simulink library "lib_controller"  (R2015a)
settings: Solver=ode45  StartTime=0.0  StopTime=10.0  RelTol=1e-3
values from neighbouring files (symbols this model uses):
  CG_0 = [0,0,0.02]'    [SetupComplete.m]
  g = 9.81    [SetupComplete.m]
  h_M = 0.064    [SetupComplete.m]
  I_BAC_0 = [ Ix,0,Ixz;0,Iy,0;Ixz,0,Iz]    [SetupComplete.m]
  l = 0.3450    (= 0.345)    [NDI_components.m]    (also in SetupComplete.m; robust_controller.m)
  m = 3.51    [SetupComplete.m]
  m_0 = 2.61    [SetupComplete.m]
  m_M = 0.300    (= 0.3)    [SetupComplete.m]
  T_sim = 0.01    [Run3Copter.m]
undefined symbols (not defined in the file or in its folder): Theta_1_roll_last, Theta_2_roll_last, Theta_3_roll_last, V_long_lastA_w_z, V_long_lastAoA, V_roll_last, V_yaw_last, W_long_lastA_w_z, W_long_lastAoA, W_roll_last, W_yaw_last
libraries: simulink x65, Adaptive_FaultTolerantControl x8, lib_controller x5, qcatlib x4, dspinverses x4, aerolibtransform2 x3, aerolib6dofsys x1
(part 5 of 10)

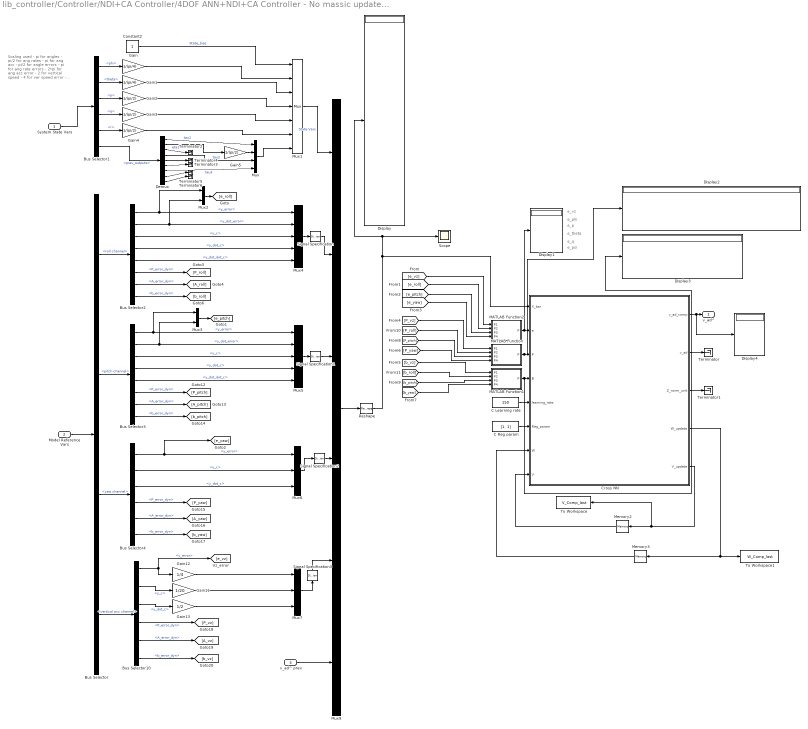
== system lib_controller/Controller/NDI+CA Controller/4DOF ANN+NDI+CA Controller - No massic update/Adaptive NN/Crossed NN ==
  note: e_vz
  note: Scaling used
      | - pi for angles
      | - pi/2 for ang rates
      | - pi for ang acc
      | - pi/2 for angle errors
      | - pi for ang rate errors
      | - 2*pi for ang acc error
      |
      | - 2 for vertical speed
      | - 4 for ver speed error
      | - 12 for vertical acc
      | - 18 for vertical acc error
  note: e_phi
  note: e_p
  note: e_theta
  note: e_q
  note: e_psi
  System State Vars : Inport
  Model Reference Vars : Inport  Port=2
  v_ad^ prev : Inport  Port=3
  Bus Selector : BusSelector  OutputSignals=roll channel,pitch channel,yaw channel,vertical acc channel
  Bus Selector1 : BusSelector  OutputSignals=phi,theta,p,q,r,prev_outputs
  Bus Selector10 : BusSelector  OutputSignals=y_error,y_c,y_dot_c,P_error_dyn,A_error_dyn,b_error_dyn
  Bus Selector2 : BusSelector  OutputSignals=y_error,y_dot_error,y_c,y_dot_c,y_dot_dot_c,P_error_dyn,A_error_dyn,b_error_dyn
  Bus Selector3 : BusSelector  OutputSignals=y_error,y_dot_error,y_c,y_dot_c,y_dot_dot_c,P_error_dyn,A_error_dyn,b_error_dyn
  Bus Selector4 : BusSelector  OutputSignals=y_error,y_c,y_dot_c,P_error_dyn,A_error_dyn,b_error_dyn
  C Learning rate : Constant  Value=150  SampleTime=T_sim
  C Reg param : Constant  Value=[1, 1]  SampleTime=T_sim
  Constant2 : Constant
  Cross NN : MATLAB Function  TreatAsAtomicUnit=on
  Demux : Demux  Outputs=9
  Display{,1..4} (5 alike) : Display
  Gain : Gain  Gain=1/(pi/4)
  Gain1 : Gain  Gain=1/(pi/4)
  Gain11 : Gain  Gain=1/20
  Gain12 : Gain  Gain=1/4
  Gain13 : Gain  Gain=1/2
  Gain{2..5} (4 alike) : Gain  Gain=1/(pi/2)
  MATLAB Function : MATLAB Function  TreatAsAtomicUnit=on
  MATLAB Function1 : MATLAB Function  TreatAsAtomicUnit=on
  MATLAB Function2 : MATLAB Function  TreatAsAtomicUnit=on
  Memory2 : Memory
  Memory3 : Memory
  Mux : Mux
  Mux1 : Mux  Inputs=7
  Mux2 : Mux  Inputs=2
  Mux3 : Mux  Inputs=2
  Mux4 : Mux  Inputs=5
  Mux5 : Mux  Inputs=5
  Mux6 : Mux  Inputs=3
  Mux7 : Mux  Inputs=3
  Mux9 : Mux  Inputs=6
  Reshape : Reshape
  Scope : Scope
      settings: SaveName=ScopeData8
  Signal Specification : SignalSpecification  Dimensions=5
  Signal Specification1 : SignalSpecification  Dimensions=5
  Signal Specification2 : SignalSpecification  Dimensions=3
  Signal Specification3 : SignalSpecification  Dimensions=3
  Terminator{,1..6} (7 alike) : Terminator
  To Workspace : ToWorkspace  VariableName=V_Comp_last  SampleTime=-1
      settings: MaxDataPoints=1
  To Workspace1 : ToWorkspace  VariableName=W_Comp_last  SampleTime=-1
      settings: MaxDataPoints=1
  v_ad^ : Outport
  wires:
  Cross NN/4(W_update) -> To Workspace1/1, Memory3/1
  Cross NN/5(V_update) -> Memory2/1, To Workspace/1
  Cross NN/2(v_ad) -> Terminator/1
  Memory3/1 -> Cross NN/7(W)
  Memory2/1 -> Cross NN/8(V)
  Cross NN/1(v_ad_comp) -> Display4/1, v_ad^/1
  C Learning rate/1 -> Cross NN/5(learning_rate)
  C Reg param/1 -> Cross NN/6(Reg_param)
  Cross NN/3(Z_norm_unit) -> Terminator1/1
  Mux9/1 -> Reshape/1
  Model Reference Vars/1 -> Bus Selector/1
  System State Vars/1 -> Bus Selector1/1
  Bus Selector1/1 -> Gain/1  "<phi>"
  Bus Selector1/2 -> Gain1/1  "<theta>"
  Bus Selector1/3 -> Gain2/1  "<p>"
  Bus Selector1/4 -> Gain3/1  "<q>"
  Bus Selector1/5 -> Gain4/1  "<r>"
  Bus Selector1/6 -> Demux/1  "<prev_outputs>"
  Gain5/1 -> Mux/2
  Mux1/1 -> Mux9/1  "State Vars"
  Mux/1 -> Mux1/7
  Gain2/1 -> Mux1/4
  Gain1/1 -> Mux1/3
  Gain3/1 -> Mux1/5
  Gain/1 -> Mux1/2
  Gain4/1 -> Mux1/6
  Constant2/1 -> Mux1/1  "State_bias"
  Bus Selector/1 -> Bus Selector2/1  "<roll channel>"
  Bus Selector2/1 -> Mux4/1, Mux2/1  "<y_error>"
  Bus Selector2/2 -> Mux4/2, Mux2/2  "<y_dot_error>"
  Bus Selector2/3 -> Mux4/3  "<y_c>"
  Bus Selector2/4 -> Mux4/4  "<y_dot_c>"
  Bus Selector2/5 -> Mux4/5  "<y_dot_dot_c>"
  Bus Selector/2 -> Bus Selector3/1  "<pitch channel>"
  Bus Selector3/1 -> Mux5/1, Mux3/1  "<y_error>"
  Bus Selector3/2 -> Mux5/2, Mux3/2  "<y_dot_error>"
  Bus Selector/3 -> Bus Selector4/1  "<yaw channel>"
  Bus Selector/4 -> Bus Selector10/1  "<vertical acc channel>"
  Bus Selector4/1 -> Mux6/1, [e_yaw]  "<y_error>"
  Mux2/1 -> [e_roll]
  Mux3/1 -> [e_pitch]
  Bus Selector2/6 -> [P_roll]  "<P_error_dyn>"
  Bus Selector2/7 -> [A_roll]  "<A_error_dyn>"
  Bus Selector2/8 -> [b_roll]  "<b_error_dyn>"
  Bus Selector10/1 -> Gain12/1, [e_vz]  "<y_error>"
  Bus Selector3/6 -> [P_pitch]  "<P_error_dyn>"
  Bus Selector3/7 -> [A_pitch]  "<A_error_dyn>"
  Bus Selector3/8 -> [b_pitch]  "<b_error_dyn>"
  Bus Selector4/4 -> [P_yaw]  "<P_error_dyn>"
  Bus Selector4/5 -> [A_yaw]  "<A_error_dyn>"
  Bus Selector4/6 -> [b_yaw]  "<b_error_dyn>"
  Bus Selector10/4 -> [P_vz]  "<P_error_dyn>"
  Bus Selector10/5 -> [A_vz]  "<A_error_dyn>"
  Bus Selector10/6 -> [b_vz]  "<b_error_dyn>"
  Bus Selector3/3 -> Mux5/3  "<y_c>"
  Bus Selector3/4 -> Mux5/4  "<y_dot_c>"
  Bus Selector3/5 -> Mux5/5  "<y_dot_dot_c>"
  Bus Selector4/2 -> Mux6/2  "<y_c>"
  Bus Selector4/3 -> Mux6/3  "<y_dot_c>"
  Bus Selector10/2 -> Gain11/1  "<y_c>"
  Bus Selector10/3 -> Gain13/1  "<y_dot_c>"
  v_ad^ prev/1 -> Mux9/6
  Reshape/1 -> Cross NN/1(X_bar), Display/1, Scope/1
  Mux5/1 -> Signal Specification1/1
  Gain12/1 -> Mux7/1
  Gain13/1 -> Mux7/3
  Gain11/1 -> Mux7/2
  Mux7/1 -> Signal Specification3/1
  MATLAB Function/1(P) -> Display2/1, Cross NN/3(P)
  [P_yaw] -> MATLAB Function/4(P4)
  [P_pitch] -> MATLAB Function/3(P3)
  [P_roll] -> MATLAB Function/2(P2)
  [P_vz] -> MATLAB Function/1(P1)
  MATLAB Function1/1(P) -> Display3/1, Cross NN/4(B)
  [b_vz] -> MATLAB Function1/1(P1)
  [b_roll] -> MATLAB Function1/2(P2)
  [b_pitch] -> MATLAB Function1/3(P3)
  [b_yaw] -> MATLAB Function1/4(P4)
  Demux/1 -> Mux/1  "tau1"
  Demux/2 -> Gain5/1  "eta1"
  Demux/4 -> Mux/3  "tau2"
  Demux/7 -> Mux/4  "tau3"
  Demux/3 -> Terminator2/1
  Demux/5 -> Terminator4/1
  Demux/6 -> Terminator3/1
  Demux/8 -> Terminator5/1
  Demux/9 -> Terminator6/1
  [e_yaw] -> MATLAB Function2/4(P4)
  [e_pitch] -> MATLAB Function2/3(P3)
  [e_roll] -> MATLAB Function2/2(P2)
  [e_vz] -> MATLAB Function2/1(P1)
  MATLAB Function2/1(P) -> Display1/1, Cross NN/2(e)
  Mux4/1 -> Signal Specification/1
  Signal Specification/1 -> Mux9/2
  Signal Specification1/1 -> Mux9/3
  Signal Specification2/1 -> Mux9/4
  Mux6/1 -> Signal Specification2/1
  Signal Specification3/1 -> Mux9/5

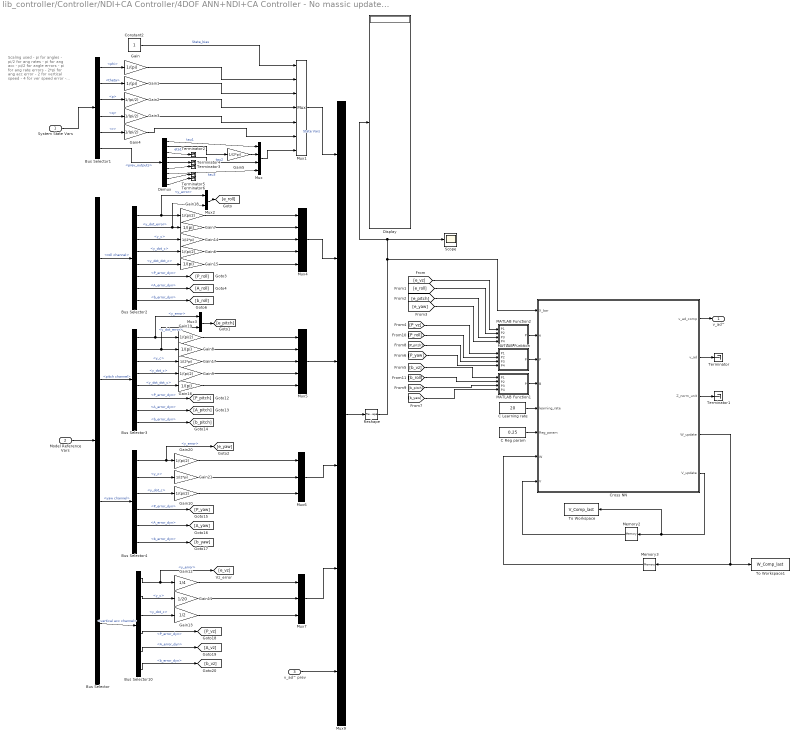
== system lib_controller/Controller/NDI+CA Controller/4DOF ANN+NDI+CA Controller - No massic update/Adaptive NN1/Complete crossed On-line (adaptive) multi-layer NN: AoA ==
  note: Scaling used
      | - pi for angles
      | - pi/2 for ang rates
      | - pi for ang acc
      | - pi/2 for angle errors
      | - pi for ang rate errors
      | - 2*pi for ang acc error
      |
      | - 2 for vertical speed
      | - 4 for ver speed error
      | - 12 for vertical acc
      | - 18 for vertical acc error
  System State Vars : Inport
  Model Reference Vars : Inport  Port=2
  v_ad^ prev : Inport  Port=3
  Bus Selector : BusSelector  OutputSignals=roll channel,pitch channel,yaw channel,vertical acc channel
  Bus Selector1 : BusSelector  OutputSignals=phi,theta,p,q,r,prev_outputs
  Bus Selector10 : BusSelector  OutputSignals=y_error,y_c,y_dot_c,P_error_dyn,A_error_dyn,b_error_dyn
  Bus Selector2 : BusSelector  OutputSignals=y_error,y_dot_error,y_c,y_dot_c,y_dot_dot_c,P_error_dyn,A_error_dyn,b_error_dyn
  Bus Selector3 : BusSelector  OutputSignals=y_error,y_dot_error,y_c,y_dot_c,y_dot_dot_c,P_error_dyn,A_error_dyn,b_error_dyn
  Bus Selector4 : BusSelector  OutputSignals=y_error,y_c,y_dot_c,P_error_dyn,A_error_dyn,b_error_dyn
  C Learning rate : Constant  Value=20  SampleTime=T_sim
  C Reg param : Constant  Value=0.25  SampleTime=T_sim
  Constant2 : Constant
  Cross NN : MATLAB Function  TreatAsAtomicUnit=on
  Demux : Demux  Outputs=9
  Display : Display
  Gain{,1,7..8,15..16} (6 alike) : Gain  Gain=1/(pi)
  Gain{2..4,6,9..10,18..20} (9 alike) : Gain  Gain=1/(pi/2)
  Gain11 : Gain  Gain=1/20
  Gain12 : Gain  Gain=1/4
  Gain13 : Gain  Gain=1/2
  Gain{5,14,17,21} (4 alike) : Gain  Gain=1/(2*pi)
  MATLAB Function : MATLAB Function  TreatAsAtomicUnit=on
  MATLAB Function1 : MATLAB Function  TreatAsAtomicUnit=on
  MATLAB Function2 : MATLAB Function  TreatAsAtomicUnit=on
  Memory2 : Memory
  Memory3 : Memory
  Mux : Mux
  Mux1 : Mux  Inputs=7
  Mux2 : Mux  Inputs=2
  Mux3 : Mux  Inputs=2
  Mux4 : Mux  Inputs=5
  Mux5 : Mux  Inputs=5
  Mux6 : Mux  Inputs=3
  Mux7 : Mux  Inputs=3
  Mux9 : Mux  Inputs=6
  Reshape : Reshape
  Scope : Scope
      settings: SaveName=ScopeData8
  Terminator{,1..6} (7 alike) : Terminator
  To Workspace : ToWorkspace  VariableName=V_Comp_last  SampleTime=-1
      settings: MaxDataPoints=1
  To Workspace1 : ToWorkspace  VariableName=W_Comp_last  SampleTime=-1
      settings: MaxDataPoints=1
  v_ad^ : Outport
  wires:
  MATLAB Function2/1(P) -> Cross NN/2(e)
  [e_vz] -> MATLAB Function2/1(P1)
  [e_roll] -> MATLAB Function2/2(P2)
  [e_pitch] -> MATLAB Function2/3(P3)
  [e_yaw] -> MATLAB Function2/4(P4)
  Demux/9 -> Terminator6/1
  Demux/8 -> Terminator5/1
  Demux/6 -> Terminator3/1
  Demux/5 -> Terminator4/1
  Demux/3 -> Terminator2/1
  Demux/7 -> Mux/4  "tau3"
  Demux/4 -> Mux/3  "tau2"
  Demux/2 -> Gain5/1  "eta1"
  Demux/1 -> Mux/1  "tau1"
  [b_yaw] -> MATLAB Function1/4(P4)
  [b_pitch] -> MATLAB Function1/3(P3)
  [b_roll] -> MATLAB Function1/2(P2)
  [b_vz] -> MATLAB Function1/1(P1)
  MATLAB Function1/1(P) -> Cross NN/4(B)
  [P_vz] -> MATLAB Function/1(P1)
  [P_roll] -> MATLAB Function/2(P2)
  [P_pitch] -> MATLAB Function/3(P3)
  [P_yaw] -> MATLAB Function/4(P4)
  MATLAB Function/1(P) -> Cross NN/3(P)
  Mux7/1 -> Mux9/5
  Gain11/1 -> Mux7/2
  Gain13/1 -> Mux7/3
  Gain12/1 -> Mux7/1
  Gain10/1 -> Mux6/3
  Gain21/1 -> Mux6/2
  Gain20/1 -> Mux6/1
  Mux6/1 -> Mux9/4
  Gain16/1 -> Mux5/5
  Gain9/1 -> Mux5/4
  Gain17/1 -> Mux5/3
  Gain8/1 -> Mux5/2
  Gain19/1 -> Mux5/1
  Mux5/1 -> Mux9/3
  Gain15/1 -> Mux4/5
  Gain6/1 -> Mux4/4
  Gain14/1 -> Mux4/3
  Gain7/1 -> Mux4/2
  Gain18/1 -> Mux4/1
  Reshape/1 -> Scope/1, Display/1, Cross NN/1(X_bar)
  Mux4/1 -> Mux9/2
  v_ad^ prev/1 -> Mux9/6
  Bus Selector10/3 -> Gain13/1  "<y_dot_c>"
  Bus Selector10/2 -> Gain11/1  "<y_c>"
  Bus Selector4/3 -> Gain10/1  "<y_dot_c>"
  Bus Selector4/2 -> Gain21/1  "<y_c>"
  Bus Selector3/5 -> Gain16/1  "<y_dot_dot_c>"
  Bus Selector3/4 -> Gain9/1  "<y_dot_c>"
  Bus Selector3/3 -> Gain17/1  "<y_c>"
  Bus Selector10/6 -> [b_vz]  "<b_error_dyn>"
  Bus Selector10/5 -> [A_vz]  "<A_error_dyn>"
  Bus Selector10/4 -> [P_vz]  "<P_error_dyn>"
  Bus Selector4/6 -> [b_yaw]  "<b_error_dyn>"
  Bus Selector4/5 -> [A_yaw]  "<A_error_dyn>"
  Bus Selector4/4 -> [P_yaw]  "<P_error_dyn>"
  Bus Selector3/8 -> [b_pitch]  "<b_error_dyn>"
  Bus Selector3/7 -> [A_pitch]  "<A_error_dyn>"
  Bus Selector3/6 -> [P_pitch]  "<P_error_dyn>"
  Bus Selector10/1 -> [e_vz], Gain12/1  "<y_error>"
  Bus Selector2/8 -> [b_roll]  "<b_error_dyn>"
  Bus Selector2/7 -> [A_roll]  "<A_error_dyn>"
  Bus Selector2/6 -> [P_roll]  "<P_error_dyn>"
  Mux3/1 -> [e_pitch]
  Mux2/1 -> [e_roll]
  Bus Selector4/1 -> [e_yaw], Gain20/1  "<y_error>"
  Bus Selector/4 -> Bus Selector10/1  "<vertical acc channel>"
  Bus Selector/3 -> Bus Selector4/1  "<yaw channel>"
  Bus Selector3/2 -> Mux3/2, Gain8/1  "<y_dot_error>"
  Bus Selector3/1 -> Mux3/1, Gain19/1  "<y_error>"
  Bus Selector/2 -> Bus Selector3/1  "<pitch channel>"
  Bus Selector2/5 -> Gain15/1  "<y_dot_dot_c>"
  Bus Selector2/4 -> Gain6/1  "<y_dot_c>"
  Bus Selector2/3 -> Gain14/1  "<y_c>"
  Bus Selector2/2 -> Gain7/1, Mux2/2  "<y_dot_error>"
  Bus Selector2/1 -> Mux2/1, Gain18/1  "<y_error>"
  Bus Selector/1 -> Bus Selector2/1  "<roll channel>"
  Constant2/1 -> Mux1/1  "State_bias"
  Gain4/1 -> Mux1/6
  Gain/1 -> Mux1/2
  Gain3/1 -> Mux1/5
  Gain1/1 -> Mux1/3
  Gain2/1 -> Mux1/4
  Mux/1 -> Mux1/7
  Mux1/1 -> Mux9/1  "State Vars"
  Gain5/1 -> Mux/2
  Bus Selector1/6 -> Demux/1  "<prev_outputs>"
  Bus Selector1/5 -> Gain4/1  "<r>"
  Bus Selector1/4 -> Gain3/1  "<q>"
  Bus Selector1/3 -> Gain2/1  "<p>"
  Bus Selector1/2 -> Gain1/1  "<theta>"
  Bus Selector1/1 -> Gain/1  "<phi>"
  System State Vars/1 -> Bus Selector1/1
  Model Reference Vars/1 -> Bus Selector/1
  Mux9/1 -> Reshape/1
  Cross NN/3(Z_norm_unit) -> Terminator1/1
  C Reg param/1 -> Cross NN/6(Reg_param)
  C Learning rate/1 -> Cross NN/5(learning_rate)
  Cross NN/1(v_ad_comp) -> v_ad^/1
  Memory2/1 -> Cross NN/8(V)
  Memory3/1 -> Cross NN/7(W)
  Cross NN/2(v_ad) -> Terminator/1
  Cross NN/5(V_update) -> To Workspace/1, Memory2/1
  Cross NN/4(W_update) -> Memory3/1, To Workspace1/1

== system lib_controller/Controller/NDI+CA Controller/4DOF ANN+NDI+CA Controller - No massic update/Control Allocation 4DOF/Control Allocation 4DOF ==
  note: Position and rate limits for
      | tricopter actuators
  note: Weights used to normalize different
      | inputs between controllers.
      | Throttle - 0 to 1
      | Servo - 0 to 2*pi
  note: Enabler override saturations and override
      | them with zero to avoid actuators being
      | locked by control allocation algorithm
  Pseudocontrol input : Inport
  Effectiveness control matrix : Inport  Port=2
  "Control allocator Completed " : qcatlib/Control allocator Completed   alg=WLS  CA_type=QP  iter_max=10  gamma=1e6  k_B=4  m_B=4  T=0.01  tol=0
  Control positions deviation Weight W1 : Constant  Value=diag(1./[1,2*pi,1,1] )
  Control rate deviation Weight W2 : Constant  Value=diag(1./[1,2*pi,1,1] )
  Demux : Demux
  Enalbe/Disable : Constant
  Error Weight Wv2 : Constant  Value=blkdiag(1, 1/(2*pi), 1/(2*pi), 1/(2*pi))
  Ground{,1..4} (5 alike) : Ground
  Mux10 : Mux  Inputs=9
  Position limits 4 DOF : Constant  Value=[ [0,-deg2rad(165),0,0]', [1,deg2rad(160),1,1]']
  Rates limits 4DOF : Constant  Value=[ [-17,-1,-17,-17]', [17,1,17,17]']*1
  Reshape1 : Reshape  OutputDimensionality=Customize  OutputDimensions=[4,4]
  Reshape2 : Reshape  OutputDimensions=[6,1]
  Terminator : Terminator
  Terminator1 : Terminator
  Unit Delay : UnitDelay  SampleTime=-1
  manual Initial saturations : Constant  Value=zeros(4,1)
  Control output : Outport  PortDimensions=9
  wires:
  Pseudocontrol input/1 -> "Control allocator Completed "/1
  Unit Delay/1 -> "Control allocator Completed "/2
  "Control allocator Completed "/1 -> Unit Delay/1, Demux/1
  Ground4/1 -> Mux10/9
  Ground3/1 -> Mux10/8
  Ground2/1 -> Mux10/6
  Ground1/1 -> Mux10/5
  Ground/1 -> Mux10/3
  Demux/4 -> Mux10/7
  Demux/3 -> Mux10/4
  Demux/2 -> Mux10/2
  Demux/1 -> Mux10/1
  Mux10/1 -> Reshape2/1
  Reshape2/1 -> Control output/1
  Enalbe/Disable/1 -> "Control allocator Completed "/11
  manual Initial saturations/1 -> "Control allocator Completed "/10
  Control rate deviation Weight W2/1 -> "Control allocator Completed "/9
  Control positions deviation Weight W1/1 -> "Control allocator Completed "/8
  Error Weight Wv2/1 -> "Control allocator Completed "/7
  Rates limits 4DOF/1 -> "Control allocator Completed "/6
  Position limits 4 DOF/1 -> "Control allocator Completed "/5
  [trimmed_input] -> "Control allocator Completed "/3
  Reshape1/1 -> "Control allocator Completed "/4
  Effectiveness control matrix/1 -> Reshape1/1
  "Control allocator Completed "/3 -> Terminator1/1
  "Control allocator Completed "/2 -> Terminator/1

== system lib_controller/Controller/NDI+CA Controller/4DOF ANN+NDI+CA Controller - No massic update/Control Allocation 4DOF/Pseudoinverse ==
  Pseudocontrol input : Inport
  Effectiveness control matrix : Inport  Port=2
  Demux : Demux
  Ground{,1..4} (5 alike) : Ground
  Mux10 : Mux  Inputs=9
  Product1 : Product  Multiplication=Matrix(*)
  Pseudoinverse : dspinverses/Pseudoinverse  wanterr=off
  Reshape1 : Reshape  OutputDimensions=[6,1]
  Control output : Outport  PortDimensions=9
  wires:
  Reshape1/1 -> Control output/1
  Pseudocontrol input/1 -> Product1/2
  Effectiveness control matrix/1 -> Pseudoinverse/1
  Pseudoinverse/1 -> Product1/1
  Mux10/1 -> Reshape1/1
  Demux/1 -> Mux10/1
  Demux/2 -> Mux10/2
  Demux/3 -> Mux10/4
  Demux/4 -> Mux10/7
  Ground/1 -> Mux10/3
  Ground1/1 -> Mux10/5
  Ground2/1 -> Mux10/6
  Ground3/1 -> Mux10/8
  Ground4/1 -> Mux10/9
  Product1/1 -> Demux/1

== system lib_controller/Controller/NDI+CA Controller/4DOF ANN+NDI+CA Controller - No massic update/On-line (adaptive) multi-layer NNs/Pitch Channel ==
  v_ad^ prev : Inport
  Long_chanel vars : Inport  Port=2
  All_meas : Inport  Port=3
  Long_learning rate : Inport  Port=4
  Long reg param : Inport  Port=5
  Long HL NN A_w_z : Subsystem  VariantControl=Long HL NN A_w_z
  Long HL NN AoA : Subsystem  VariantControl=Long HL NN AoA
  v_ad_comp : Outport

== system lib_controller/Controller/NDI+CA Controller/4DOF ANN+NDI+CA Controller - No massic update/On-line (adaptive) multi-layer NNs/Roll Channel ==
  v_ad^ prev : Inport
  p_chanel vars : Inport  Port=2
  All_meas : Inport  Port=3
  Roll_learning rate : Inport  Port=4
  Roll reg param : Inport  Port=5
  Roll 1HL NN : Subsystem  VariantControl=Roll 1HL NN
  Roll 2HL NN : Subsystem  VariantControl=Roll 2HL NN
  v_ad_comp : Outport

== system lib_controller/Controller/NDI+CA Controller/4DOF ANN+NDI+CA Controller - No massic update/On-line (adaptive) multi-layer NNs/Yaw Channel ==
  v_ad^ prev : Inport
  Yaw_chanel vars : Inport  Port=2
  All_meas : Inport  Port=3
  Yaw_learning rate : Inport  Port=4
  Yaw reg param : Inport  Port=5
  Yaw HL NN : Subsystem  VariantControl=Yaw HL NN
  v_ad_comp : Outport

== system lib_controller/Controller/NDI+CA Controller/4DOF NDI+CA Controller - No massic update/Control Allocation 4DOF/Control Allocation 4DOF ==
  note: Enabler override saturations and override
      | them with zero to avoid actuators being
      | locked by control allocation algorithm
  note: Weights used to normalize different
      | inputs between controllers.
      | Throttle - 0 to 1
      | Servo - 0 to 2*pi
  note: Position and rate limits for
      | tricopter actuators
  Pseudocontrol input : Inport
  Effectiveness control matrix : Inport  Port=2
  "Control allocator Completed " : qcatlib/Control allocator Completed   alg=WLS  CA_type=QP  iter_max=10  gamma=1e6  k_B=4  m_B=4  T=0.01  tol=0
  Control desired (0 to minimize control effort) : Constant  Value=zeros(1,4)
  Control positions deviation Weight W1 : Constant  Value=diag(1./[1,2*pi,1,1] )
  Control rate deviation Weight W2 : Constant  Value=diag(1./[1,2*pi,1,1] )
  Demux : Demux
  Enalbe/Disable : Constant
  Error Weight Wv2 : Constant  Value=blkdiag(1, 1/(2*pi), 1/(2*pi), 1/(2*pi))
  Ground{,1..4} (5 alike) : Ground
  Mux10 : Mux  Inputs=9
  Position limits 4 DOF : Constant  Value=[ [0,-deg2rad(165),0,0]', [1,deg2rad(160),1,1]']
  Rates limits 4DOF : Constant  Value=[ [-17,-1,-17,-17]', [17,1,17,17]']*1
  Reshape1 : Reshape  OutputDimensionality=Customize  OutputDimensions=[4,4]
  Reshape2 : Reshape  OutputDimensions=[6,1]
  Terminator : Terminator
  Terminator1 : Terminator
  Unit Delay : UnitDelay  SampleTime=-1
  manual Initial saturations : Constant  Value=zeros(4,1)
  Control output : Outport  PortDimensions=9
  wires:
  "Control allocator Completed "/2 -> Terminator/1
  "Control allocator Completed "/3 -> Terminator1/1
  Effectiveness control matrix/1 -> Reshape1/1
  Reshape1/1 -> "Control allocator Completed "/4
  Control desired (0 to minimize control effort)/1 -> "Control allocator Completed "/3
  Position limits 4 DOF/1 -> "Control allocator Completed "/5
  Rates limits 4DOF/1 -> "Control allocator Completed "/6
  Error Weight Wv2/1 -> "Control allocator Completed "/7
  Control positions deviation Weight W1/1 -> "Control allocator Completed "/8
  Control rate deviation Weight W2/1 -> "Control allocator Completed "/9
  manual Initial saturations/1 -> "Control allocator Completed "/10
  Enalbe/Disable/1 -> "Control allocator Completed "/11
  Reshape2/1 -> Control output/1
  Mux10/1 -> Reshape2/1
  Demux/1 -> Mux10/1
  Demux/2 -> Mux10/2
  Demux/3 -> Mux10/4
  Demux/4 -> Mux10/7
  Ground/1 -> Mux10/3
  Ground1/1 -> Mux10/5
  Ground2/1 -> Mux10/6
  Ground3/1 -> Mux10/8
  Ground4/1 -> Mux10/9
  "Control allocator Completed "/1 -> Demux/1, Unit Delay/1
  Unit Delay/1 -> "Control allocator Completed "/2
  Pseudocontrol input/1 -> "Control allocator Completed "/1

== system lib_controller/Controller/NDI+CA Controller/4DOF NDI+CA Controller - No massic update/Control Allocation 4DOF/Pseudoinverse ==
  Pseudocontrol input : Inport
  Effectiveness control matrix : Inport  Port=2
  Demux : Demux
  Ground{,1..4} (5 alike) : Ground
  Mux10 : Mux  Inputs=9
  Product1 : Product  Multiplication=Matrix(*)
  Pseudoinverse : dspinverses/Pseudoinverse  wanterr=off
  Reshape1 : Reshape  OutputDimensions=[6,1]
  Control output : Outport  PortDimensions=9
  wires:
  Product1/1 -> Demux/1
  Ground4/1 -> Mux10/9
  Ground3/1 -> Mux10/8
  Ground2/1 -> Mux10/6
  Ground1/1 -> Mux10/5
  Ground/1 -> Mux10/3
  Demux/4 -> Mux10/7
  Demux/3 -> Mux10/4
  Demux/2 -> Mux10/2
  Demux/1 -> Mux10/1
  Mux10/1 -> Reshape1/1
  Pseudoinverse/1 -> Product1/1
  Effectiveness control matrix/1 -> Pseudoinverse/1
  Pseudocontrol input/1 -> Product1/2
  Reshape1/1 -> Control output/1

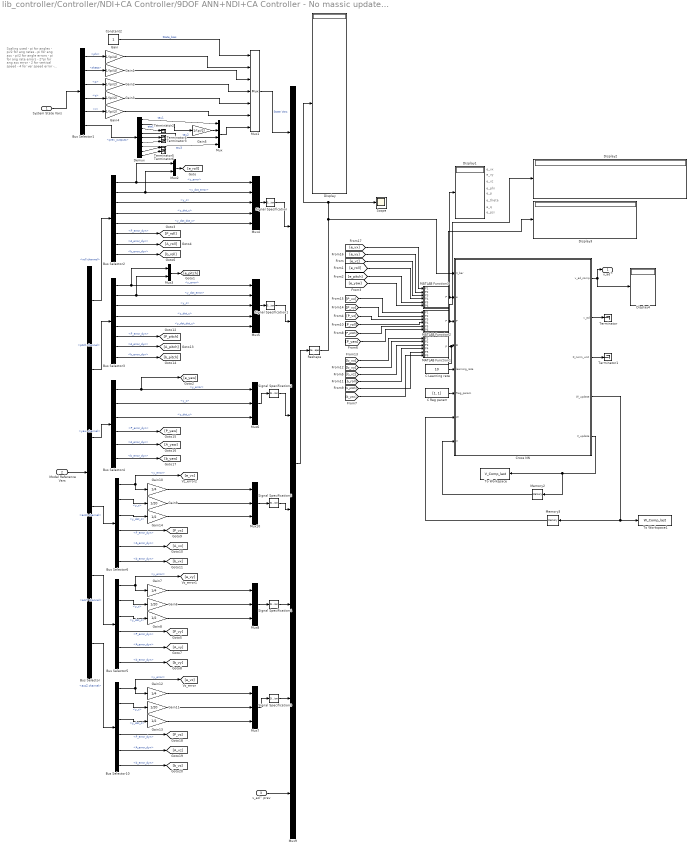
== system lib_controller/Controller/NDI+CA Controller/9DOF ANN+NDI+CA Controller - No massic update/Adaptive NN/Crossed NN ==
  note: e_vx
  note: e_vy
  note: e_vz
  note: Scaling used
      | - pi for angles
      | - pi/2 for ang rates
      | - pi for ang acc
      | - pi/2 for angle errors
      | - pi for ang rate errors
      | - 2*pi for ang acc error
      |
      | - 2 for vertical speed
      | - 4 for ver speed error
      | - 12 for vertical acc
      | - 18 for vertical acc error
  note: e_phi
  note: e_p
  note: e_theta
  note: e_q
  note: e_psi
  System State Vars : Inport
  Model Reference Vars : Inport  Port=2
  v_ad^ prev : Inport  Port=3
  Bus Selector : BusSelector  OutputSignals=roll channel,pitch channel,yaw channel,accX channel,accY channel,accZ channel
  Bus Selector1 : BusSelector  OutputSignals=phi,theta,p,q,r,prev_outputs
  Bus Selector{4..6,10} (4 alike) : BusSelector  OutputSignals=y_error,y_c,y_dot_c,P_error_dyn,A_error_dyn,b_error_dyn
  Bus Selector2 : BusSelector  OutputSignals=y_error,y_dot_error,y_c,y_dot_c,y_dot_dot_c,P_error_dyn,A_error_dyn,b_error_dyn
  Bus Selector3 : BusSelector  OutputSignals=y_error,y_dot_error,y_c,y_dot_c,y_dot_dot_c,P_error_dyn,A_error_dyn,b_error_dyn
  C Learning rate : Constant  Value=10  SampleTime=T_sim
  C Reg param : Constant  Value=[1, 1]  SampleTime=T_sim
  Constant2 : Constant
  Cross NN : MATLAB Function  TreatAsAtomicUnit=on
  Demux : Demux  Outputs=9
  Display{,1..4} (5 alike) : Display
  Gain : Gain  Gain=1/(pi/4)
  Gain1 : Gain  Gain=1/(pi/4)
  Gain10 : Gain  Gain=1/4
  Gain11 : Gain  Gain=1/20
  Gain12 : Gain  Gain=1/4
  Gain13 : Gain  Gain=1/2
  Gain14 : Gain  Gain=1/2
  Gain{2..5} (4 alike) : Gain  Gain=1/(pi/2)
  Gain6 : Gain  Gain=1/20
  Gain7 : Gain  Gain=1/4
  Gain8 : Gain  Gain=1/2
  Gain9 : Gain  Gain=1/20
  MATLAB Function1 : MATLAB Function  TreatAsAtomicUnit=on
  MATLAB Function2 : MATLAB Function  TreatAsAtomicUnit=on
  MATLAB Function3 : MATLAB Function  TreatAsAtomicUnit=on
  Memory2 : Memory
  Memory3 : Memory
  Mux : Mux
  Mux1 : Mux  Inputs=7
  Mux{6..8,10} (4 alike) : Mux  Inputs=3
  Mux2 : Mux  Inputs=2
  Mux3 : Mux  Inputs=2
  Mux4 : Mux  Inputs=5
  Mux5 : Mux  Inputs=5
  Mux9 : Mux  Inputs=8
  Reshape : Reshape
  Scope : Scope
      settings: SaveName=ScopeData8
  Signal Specification : SignalSpecification  Dimensions=5
  Signal Specification1 : SignalSpecification  Dimensions=5
  Signal Specification{2..5} (4 alike) : SignalSpecification  Dimensions=3
  Terminator{,1..6} (7 alike) : Terminator
  To Workspace : ToWorkspace  VariableName=V_Comp_last  SampleTime=-1
      settings: MaxDataPoints=1
  To Workspace1 : ToWorkspace  VariableName=W_Comp_last  SampleTime=-1
      settings: MaxDataPoints=1
  v_ad^ : Outport
  wires:
  MATLAB Function1/1(P) -> Display3/1, Cross NN/4(B)
  [e_yaw] -> MATLAB Function3/6(P6)
  [e_pitch] -> MATLAB Function3/5(P5)
  [e_roll] -> MATLAB Function3/4(P4)
  [e_vz] -> MATLAB Function3/3(P3)
  [e_vx] -> MATLAB Function3/1(P1)
  [e_vy] -> MATLAB Function3/2(P2)
  [P_vx] -> MATLAB Function2/1(P1)
  [P_yaw] -> MATLAB Function2/6(P6)
  [P_vy] -> MATLAB Function2/2(P2)
  [P_pitch] -> MATLAB Function2/5(P5)
  [P_vz] -> MATLAB Function2/3(P3)
  [P_roll] -> MATLAB Function2/4(P4)
  [b_vz] -> MATLAB Function1/3(P3)
  [b_vy] -> MATLAB Function1/2(P2)
  [b_yaw] -> MATLAB Function1/6(P6)
  [b_pitch] -> MATLAB Function1/5(P5)
  [b_roll] -> MATLAB Function1/4(P4)
  [b_vx] -> MATLAB Function1/1(P1)
  Signal Specification3/1 -> Mux9/7
  Signal Specification4/1 -> Mux9/6
  Signal Specification5/1 -> Mux9/5
  Bus Selector/4 -> Bus Selector6/1  "<accX channel>"
  Bus Selector6/1 -> Gain10/1, [e_vx]  "<y_error>"
  Bus Selector6/4 -> [P_vx]  "<P_error_dyn>"
  Bus Selector6/5 -> [A_vx]  "<A_error_dyn>"
  Bus Selector6/6 -> [b_vx]  "<b_error_dyn>"
  Bus Selector6/2 -> Gain9/1  "<y_c>"
  Bus Selector6/3 -> Gain14/1  "<y_dot_c>"
  Gain10/1 -> Mux10/1
  Gain14/1 -> Mux10/3
  Gain9/1 -> Mux10/2
  Mux10/1 -> Signal Specification5/1
  Bus Selector/5 -> Bus Selector5/1  "<accY channel>"
  Bus Selector5/1 -> [e_vy], Gain7/1  "<y_error>"
  Bus Selector5/4 -> [P_vy]  "<P_error_dyn>"
  Bus Selector5/5 -> [A_vy]  "<A_error_dyn>"
  Bus Selector5/6 -> [b_vy]  "<b_error_dyn>"
  Bus Selector5/2 -> Gain6/1  "<y_c>"
  Bus Selector5/3 -> Gain8/1  "<y_dot_c>"
  Gain7/1 -> Mux8/1
  Gain8/1 -> Mux8/3
  Gain6/1 -> Mux8/2
  Mux8/1 -> Signal Specification4/1
  v_ad^ prev/1 -> Mux9/8
  Cross NN/4(W_update) -> To Workspace1/1, Memory3/1
  Cross NN/5(V_update) -> To Workspace/1, Memory2/1
  Cross NN/2(v_ad) -> Terminator/1
  Memory3/1 -> Cross NN/7(W)
  Memory2/1 -> Cross NN/8(V)
  Cross NN/1(v_ad_comp) -> Display4/1, v_ad^/1
  C Learning rate/1 -> Cross NN/5(learning_rate)
  C Reg param/1 -> Cross NN/6(Reg_param)
  Cross NN/3(Z_norm_unit) -> Terminator1/1
  Mux9/1 -> Reshape/1
  Model Reference Vars/1 -> Bus Selector/1
  System State Vars/1 -> Bus Selector1/1
  Bus Selector1/1 -> Gain/1  "<phi>"
  Bus Selector1/2 -> Gain1/1  "<theta>"
  Bus Selector1/3 -> Gain2/1  "<p>"
  Bus Selector1/4 -> Gain3/1  "<q>"
  Bus Selector1/5 -> Gain4/1  "<r>"
  Bus Selector1/6 -> Demux/1  "<prev_outputs>"
  Gain5/1 -> Mux/2
  Mux1/1 -> Mux9/1  "State Vars"
  Mux/1 -> Mux1/7
  Gain2/1 -> Mux1/4
  Gain1/1 -> Mux1/3
  Gain3/1 -> Mux1/5
  Gain/1 -> Mux1/2
  Gain4/1 -> Mux1/6
  Constant2/1 -> Mux1/1  "State_bias"
  Bus Selector/1 -> Bus Selector2/1  "<roll channel>"
  Bus Selector2/1 -> Mux4/1, Mux2/1  "<y_error>"
  Bus Selector2/2 -> Mux4/2, Mux2/2  "<y_dot_error>"
  Bus Selector2/3 -> Mux4/3  "<y_c>"
  Bus Selector2/4 -> Mux4/4  "<y_dot_c>"
  Bus Selector2/5 -> Mux4/5  "<y_dot_dot_c>"
  Bus Selector/2 -> Bus Selector3/1  "<pitch channel>"
  Bus Selector3/1 -> Mux5/1, Mux3/1  "<y_error>"
  Bus Selector3/2 -> Mux5/2, Mux3/2  "<y_dot_error>"
  Bus Selector/3 -> Bus Selector4/1  "<yaw channel>"
  Bus Selector/6 -> Bus Selector10/1  "<accZ channel>"
  Bus Selector4/1 -> Mux6/1, [e_yaw]  "<y_error>"
  Mux2/1 -> [e_roll]
  Mux3/1 -> [e_pitch]
  Bus Selector2/6 -> [P_roll]  "<P_error_dyn>"
  Bus Selector2/7 -> [A_roll]  "<A_error_dyn>"
  Bus Selector2/8 -> [b_roll]  "<b_error_dyn>"
  Bus Selector10/1 -> Gain12/1, [e_vz]  "<y_error>"
  Bus Selector3/6 -> [P_pitch]  "<P_error_dyn>"
  Bus Selector3/7 -> [A_pitch]  "<A_error_dyn>"
  Bus Selector3/8 -> [b_pitch]  "<b_error_dyn>"
  Bus Selector4/4 -> [P_yaw]  "<P_error_dyn>"
  Bus Selector4/5 -> [A_yaw]  "<A_error_dyn>"
  Bus Selector4/6 -> [b_yaw]  "<b_error_dyn>"
  Bus Selector10/4 -> [P_vz]  "<P_error_dyn>"
  Bus Selector10/5 -> [A_vz]  "<A_error_dyn>"
  Bus Selector10/6 -> [b_vz]  "<b_error_dyn>"
  Bus Selector3/3 -> Mux5/3  "<y_c>"
  Bus Selector3/4 -> Mux5/4  "<y_dot_c>"
  Bus Selector3/5 -> Mux5/5  "<y_dot_dot_c>"
  Bus Selector4/2 -> Mux6/2  "<y_c>"
  Bus Selector4/3 -> Mux6/3  "<y_dot_c>"
  Bus Selector10/2 -> Gain11/1  "<y_c>"
  Bus Selector10/3 -> Gain13/1  "<y_dot_c>"
  Reshape/1 -> Cross NN/1(X_bar), Display/1, Scope/1
  Mux5/1 -> Signal Specification1/1
  Gain12/1 -> Mux7/1
  Gain13/1 -> Mux7/3
  Gain11/1 -> Mux7/2
  Mux7/1 -> Signal Specification3/1
  MATLAB Function2/1(P) -> Cross NN/3(P), Display2/1
  Demux/1 -> Mux/1  "tau1"
  Demux/2 -> Gain5/1  "eta1"
  Demux/4 -> Mux/3  "tau2"
  Demux/7 -> Mux/4  "tau3"
  Demux/3 -> Terminator2/1
  Demux/5 -> Terminator4/1
  Demux/6 -> Terminator3/1
  Demux/8 -> Terminator5/1
  Demux/9 -> Terminator6/1
  MATLAB Function3/1(P) -> Cross NN/2(e), Display1/1
  Mux4/1 -> Signal Specification/1
  Signal Specification/1 -> Mux9/2
  Signal Specification1/1 -> Mux9/3
  Signal Specification2/1 -> Mux9/4
  Mux6/1 -> Signal Specification2/1

== system lib_controller/Controller/NDI+CA Controller/9DOF ANN+NDI+CA Controller - No massic update/Control Allocation 9DOF/Control Allocation 9DOF ==
  note: Enabler override saturations and override
      | them with zero to avoid actuators being
      | locked by control allocation algorithm
  note: Weights used to normalize different
      | inputs between controllers.
      | Throttle - 0 to 1
      | Servo - 0 to 2*pi
  note: Position and rate limits for
      | tricopter actuators
  Pseudocontrol input : Inport
  Effectiveness control matrix : Inport  Port=2
  "Control allocator Completed " : qcatlib/Control allocator Completed   alg=WLS  CA_type=QP  iter_max=4  gamma=1e6  k_B=6  m_B=9  T=0.01  tol=0
  Control desired (0 to minimize control effort) : Constant  Value=zeros(1,9)
  Control desired (Timmed 9DOF) : Constant  Value=[0.6049, -0.7465,-0.07355,0.6044,-0.7422,0.4171,0.6044,0.5941,0.417]
  Control positions deviation Weight W1 : Constant  Value=diag(1./[1,2*pi,2*pi,1,2*pi,2*pi,1,2*pi,2*pi] )
  Control rate deviation Weight W2 : Constant  Value=diag(1./[1,2*pi,2*pi,1,2*pi,2*pi,1,2*pi,2*pi] )
  Enalbe/Disable : Constant
  Error Weight Wv2 : Constant  Value=blkdiag(1,1,1, 1/(2*pi), 1/(2*pi), 1/(2*pi))
  Position limits 9DOF : Constant  Value=[ [0,-deg2rad(165),-deg2rad(90),0,-deg2rad(165),-deg2rad(15),0,-deg2rad(165),-deg2rad(90)]', [1,deg2rad(165),deg2rad(15),1,deg2rad(165),deg2rad(90),1,deg2rad(165),deg2rad(15)]']
  Rates limits 9DOF : Constant  Value=[ [-17,-1,-1,-17,-1,-1,-17,-1,-1]', [17,1,1,17,1,1,17,1,1]']*1
  Reshape1 : Reshape  OutputDimensionality=Customize  OutputDimensions=[6,9]
  Reshape2 : Reshape  OutputDimensions=[6,1]
  Terminator : Terminator
  Terminator1 : Terminator
  Unit Delay : UnitDelay  SampleTime=-1
  manual Initial saturations : Constant  Value=zeros(9,1)
  Control output : Outport  PortDimensions=9
  wires:
  "Control allocator Completed "/2 -> Terminator/1
  "Control allocator Completed "/3 -> Terminator1/1
  Effectiveness control matrix/1 -> Reshape1/1
  Reshape1/1 -> "Control allocator Completed "/4
  Position limits 9DOF/1 -> "Control allocator Completed "/5
  Rates limits 9DOF/1 -> "Control allocator Completed "/6
  Error Weight Wv2/1 -> "Control allocator Completed "/7
  Control positions deviation Weight W1/1 -> "Control allocator Completed "/8
  Control rate deviation Weight W2/1 -> "Control allocator Completed "/9
  manual Initial saturations/1 -> "Control allocator Completed "/10
  Enalbe/Disable/1 -> "Control allocator Completed "/11
  Reshape2/1 -> Control output/1
  "Control allocator Completed "/1 -> Reshape2/1, Unit Delay/1
  Unit Delay/1 -> "Control allocator Completed "/2
  Pseudocontrol input/1 -> "Control allocator Completed "/1
  Control desired (Timmed 9DOF)/1 -> "Control allocator Completed "/3

== system lib_controller/Controller/NDI+CA Controller/9DOF ANN+NDI+CA Controller - No massic update/Control Allocation 9DOF/Pseudoinverse 9DOF ==
  Pseudocontrol input : Inport
  Effectiveness control matrix : Inport  Port=2
  Product1 : Product  Multiplication=Matrix(*)
  Pseudoinverse : dspinverses/Pseudoinverse  wanterr=off
  Reshape1 : Reshape  OutputDimensions=[6,1]
  Control output : Outport  PortDimensions=9
  wires:
  Product1/1 -> Reshape1/1
  Pseudoinverse/1 -> Product1/1
  Effectiveness control matrix/1 -> Pseudoinverse/1
  Pseudocontrol input/1 -> Product1/2
  Reshape1/1 -> Control output/1

== system lib_controller/Controller/NDI+CA Controller/4DOF ANN+NDI+CA Controller - No massic update/On-line (adaptive) multi-layer NNs/Pitch Channel/Long HL NN A_w_z ==
  note: Be careful with dimensions of inputs!!!
      | NORMALIZATION!!!
  v_ad^ prev : Inport
  Long_chanel vars : Inport  Port=2
  All_meas : Inport  Port=3
  Long_learning rate : Inport  Port=4
  Long reg param : Inport  Port=5
  Bus Selector1 : BusSelector  OutputSignals=A_chanel vars.A_err,q_chanel_vars.q_err,A_chanel vars.A_sf,A_chanel vars.A_sf_dot,q_chanel_vars.q_sf_dot,A_chanel vars.K_b_A,q_chanel_vars.K_b_q,A_chanel vars.FactorF
  Bus Selector2 : BusSelector  OutputSignals=signal1.Alt meas (m),signal2.Mach
  Constant : Constant
  Constant1 : Constant  Value=[0;1]
  Divide : Product  Inputs=**
  Long NN : MATLAB Function  TreatAsAtomicUnit=on
  Memory2 : Memory  X0=V_long_lastA_w_z
  Memory3 : Memory  X0=W_long_lastA_w_z
  Mux : Mux  Inputs=10
  Mux1 : Mux  Inputs=2
  Mux2 : Mux  Inputs=2
  Scope : Scope
      settings: YMin=0  YMax=0.003  SaveName=ScopeData13
  Terminator : Terminator
  Terminator1 : Terminator
  To Workspace : ToWorkspace  VariableName=V_long_lastA_w_z  SampleTime=-1
      settings: MaxDataPoints=1
  To Workspace1 : ToWorkspace  VariableName=W_long_lastA_w_z  SampleTime=-1
      settings: MaxDataPoints=1
  dim-less : Gain  Gain=T_sim
  dim-less1 : Gain  Gain=T_sim^2
  scaling : Gain  Gain=1/15000
  scaling1 : Gain  Gain=1/(9*9.81)
  scaling2 : Gain  Gain=1/(9*9.81)
  scaling3 : Gain  Gain=1/(9*9.81)
  v_ad_comp : Outport
  wires:
  Long NN/2(v_ad) -> Terminator/1
  Long NN/5(V_update) -> To Workspace/1, Memory2/1
  v_ad^ prev/1 -> Mux/10
  [Ks] -> Long NN/4(Ks)
  Constant1/1 -> Long NN/5(B)
  Memory3/1 -> Long NN/8(W)
  Memory2/1 -> Long NN/9(V)
  Long NN/4(W_update) -> To Workspace1/1, Memory3/1
  Long NN/1(v_ad_comp) -> v_ad_comp/1
  Mux/1 -> Scope/1, Long NN/1(X_bar)
  Long_chanel vars/1 -> Bus Selector1/1
  Long_learning rate/1 -> Long NN/6(Long_learnign_rate)
  Long reg param/1 -> Long NN/7(Long_reg_param)
  Constant/1 -> Mux/1
  All_meas/1 -> Bus Selector2/1
  Bus Selector2/1 -> scaling/1  "<Alt meas (m)>"
  Divide/1 -> Mux/4
  scaling/1 -> Mux/2
  Bus Selector2/2 -> Mux/3, Divide/2, Divide/1  "<Mach>"
  Bus Selector1/1 -> Mux1/1, scaling2/1  "<A_err>"
  Bus Selector1/2 -> Mux1/2, Mux/6  "<q_err>"
  Bus Selector1/3 -> scaling1/1  "<A_sf>"
  Bus Selector1/4 -> dim-less/1  "<A_sf_dot>"
  Bus Selector1/5 -> dim-less1/1  "<q_sf_dot>"
  Mux1/1 -> Long NN/2(e)  "e"
  Bus Selector1/7 -> Mux2/2  "<K_b_q>"
  Bus Selector1/6 -> Mux2/1  "<K_b_A>"
  Mux2/1 -> [Ks]
  Bus Selector1/8 -> Long NN/3(F)  "<FactorF>"
  scaling2/1 -> Mux/5
  scaling1/1 -> Mux/7
  scaling3/1 -> Mux/8
  Long NN/3(Z_norm_unit) -> Terminator1/1
  dim-less/1 -> scaling3/1
  dim-less1/1 -> Mux/9

== system lib_controller/Controller/NDI+CA Controller/4DOF ANN+NDI+CA Controller - No massic update/On-line (adaptive) multi-layer NNs/Pitch Channel/Long HL NN AoA ==
  note: Be careful with dimensions of inputs!!!
      | NORMALIZATION!!!
  v_ad^ prev : Inport
  Long_chanel vars : Inport  Port=2
  All_meas : Inport  Port=3
  Long_learning rate : Inport  Port=4
  Long reg param : Inport  Port=5
  Bus Selector1 : BusSelector  OutputSignals=alpha_chanel vars.alpha_err,q_chanel_vars.q_err,alpha_chanel vars.alpha_sf,alpha_chanel vars.alpha_sf_dot,q_chanel_vars.q_sf_dot,alpha_chanel vars.K_b_alpha,q_chanel_vars.K_b_q
  Bus Selector2 : BusSelector  OutputSignals=signal1.Alt meas (m),signal2.Mach
  Constant : Constant
  Constant1 : Constant  Value=[0;1]
  Display : Display
  Divide : Product  Inputs=**
  Gain : Gain  Gain=1/15000
  Long NN : MATLAB Function  TreatAsAtomicUnit=on
  Memory2 : Memory  X0=V_long_lastAoA
  Memory3 : Memory  X0=W_long_lastAoA
  Mux : Mux  Inputs=10
  Mux1 : Mux  Inputs=2
  Mux2 : Mux  Inputs=2
  Scope : Scope
      settings: YMin=-0.7  YMax=1  SaveName=ScopeData18
  Terminator : Terminator
  Terminator1 : Terminator
  To Workspace : ToWorkspace  VariableName=V_long_lastAoA  SampleTime=-1
      settings: MaxDataPoints=1
  To Workspace1 : ToWorkspace  VariableName=W_long_lastAoA  SampleTime=-1
      settings: MaxDataPoints=1
  dem-less : Gain  Gain=T_sim
  dem-less1 : Gain  Gain=T_sim^2
  v_ad_comp : Outport
  wires:
  Long NN/2(v_ad) -> Terminator/1
  Long NN/5(V_update) -> To Workspace/1, Memory2/1
  v_ad^ prev/1 -> Mux/10
  [Ks] -> Long NN/3(Ks)
  Constant1/1 -> Long NN/4(B)
  Memory3/1 -> Long NN/7(W)
  Memory2/1 -> Long NN/8(V)
  Long NN/4(W_update) -> To Workspace1/1, Memory3/1
  Long NN/1(v_ad_comp) -> v_ad_comp/1
  Long_chanel vars/1 -> Bus Selector1/1
  Long_learning rate/1 -> Long NN/5(Long_learnign_rate)
  Long reg param/1 -> Long NN/6(Long_reg_param)
  Constant/1 -> Mux/1
  All_meas/1 -> Bus Selector2/1
  Bus Selector2/1 -> Gain/1  "<Alt meas (m)>"
  Divide/1 -> Mux/4
  Gain/1 -> Mux/2
  Bus Selector2/2 -> Mux/3, Divide/2, Divide/1  "<Mach>"
  Bus Selector1/1 -> Mux1/1, Mux/5  "<alpha_err>"
  Bus Selector1/2 -> Mux1/2, Mux/6  "<q_err>"
  Bus Selector1/3 -> Mux/7  "<alpha_sf>"
  Bus Selector1/4 -> dem-less/1  "<alpha_sf_dot>"
  Bus Selector1/5 -> dem-less1/1  "<q_sf_dot>"
  Mux1/1 -> Long NN/2(e)  "e"
  Bus Selector1/7 -> Mux2/2  "<K_b_q>"
  Bus Selector1/6 -> Mux2/1  "<K_b_alpha>"
  Mux2/1 -> [Ks]
  Long NN/3(Z_norm_unit) -> Terminator1/1
  Mux/1 -> Scope/1, Display/1, Long NN/1(X_bar)
  dem-less/1 -> Mux/8
  dem-less1/1 -> Mux/9

== system lib_controller/Controller/NDI+CA Controller/4DOF ANN+NDI+CA Controller - No massic update/On-line (adaptive) multi-layer NNs/Roll Channel/Roll 1HL NN ==
  note: Be careful with dimensions of inputs!!!
      | NORMALIZATION!!!
  v_ad^ prev : Inport
  p_chanel vars : Inport  Port=2
  All_meas : Inport  Port=3
  Roll_learning rate : Inport  Port=4
  Roll reg param : Inport  Port=5
  Bus Selector1 : BusSelector  OutputSignals=p_err,p_sf,p_sf_dot,K_b_p
  Bus Selector2 : BusSelector  OutputSignals=signal1.Alt meas (m),signal2.Mach,signal1.AoA meas (rad),signal1.SS meas (rad),signal1.omega_b meas (rad/s)
  Constant : Constant
  Constant1 : Constant
  Constant2 : Constant
  Display : Display
  Divide : Product  Inputs=**
  Divide1 : Product  Inputs=**
  Divide2 : Product  Inputs=*/
  Memory2 : Memory  X0=V_roll_last
  Memory3 : Memory  X0=W_roll_last
  Mux : Mux  Inputs=12
  Roll NN : MATLAB Function  TreatAsAtomicUnit=on
  Scope : Scope
      settings: YMin=-0.5  YMax=6  SaveName=ScopeData15
  Selector : Selector  InputPortWidth=3  Indices=3
  Terminator : Terminator
  Terminator1 : Terminator
  To Workspace : ToWorkspace  VariableName=V_roll_last  SampleTime=-1
      settings: MaxDataPoints=1
  To Workspace1 : ToWorkspace  VariableName=W_roll_last  SampleTime=-1
      settings: MaxDataPoints=1
  dem-less : Gain  Gain=T_sim
  dim-less : Gain  Gain=1/15000
  v_ad_comp : Outport
  wires:
  Constant2/1 -> Divide2/1
  Bus Selector1/4 -> Divide2/2  "<K_b_p>"
  Divide2/1 -> [P]
  Roll NN/2(v_ad) -> Terminator/1
  Roll NN/5(V_update) -> To Workspace/1, Memory2/1
  v_ad^ prev/1 -> Mux/12
  [P] -> Roll NN/3(P)
  Constant1/1 -> Roll NN/4(B)
  Memory3/1 -> Roll NN/7(W)
  Memory2/1 -> Roll NN/8(V)
  Roll NN/4(W_update) -> To Workspace1/1, Memory3/1
  Roll NN/1(v_ad_comp) -> v_ad_comp/1
  Mux/1 -> Roll NN/1(X_bar), Scope/1, Display/1
  Bus Selector1/1 -> Mux/9, Roll NN/2(e)  "<p_err>"
  Bus Selector1/3 -> dem-less/1  "<p_sf_dot>"
  Bus Selector1/2 -> Mux/10  "<p_sf>"
  p_chanel vars/1 -> Bus Selector1/1
  Roll_learning rate/1 -> Roll NN/5(Roll_learnign_rate)
  Roll reg param/1 -> Roll NN/6(Roll_reg_param)
  Constant/1 -> Mux/1
  All_meas/1 -> Bus Selector2/1
  Bus Selector2/1 -> dim-less/1  "<Alt meas (m)>"
  Divide/1 -> Mux/4
  Bus Selector2/3 -> Divide1/2, Divide1/1, Mux/5  "<AoA meas (rad)>"
  Divide1/1 -> Mux/6
  Bus Selector2/4 -> Mux/7  "<SS meas (rad)>"
  dim-less/1 -> Mux/2
  Bus Selector2/5 -> Selector/1  "<omega_b meas (rad/s)>"
  Selector/1 -> Mux/8
  Bus Selector2/2 -> Divide/2, Divide/1, Mux/3  "<Mach>"
  Roll NN/3(Z_norm_unit) -> Terminator1/1
  dem-less/1 -> Mux/11

== system lib_controller/Controller/NDI+CA Controller/4DOF ANN+NDI+CA Controller - No massic update/On-line (adaptive) multi-layer NNs/Roll Channel/Roll 2HL NN ==
  note: Be careful with dimensions of inputs!!!
      | NORMALIZATION!!!
  v_ad^ prev : Inport
  p_chanel vars : Inport  Port=2
  All_meas : Inport  Port=3
  Roll_learning rate : Inport  Port=4
  Roll reg param : Inport  Port=5
  " " : ToWorkspace  VariableName=Theta_3_roll_last  SampleTime=-1
      settings: MaxDataPoints=1
  "  " : Memory  X0=Theta_3_roll_last
  "   " : Memory  X0=Theta_2_roll_last
  B : Constant
  Bus Selector1 : BusSelector  OutputSignals=p_err,p_sf,p_sf_dot,K_b_p
  Bus Selector2 : BusSelector  OutputSignals=signal1.Alt meas (m),signal2.Mach,signal1.AoA meas (rad),signal1.SS meas (rad),signal1.omega_b meas (rad/s)
  Constant : Constant
  Constant2 : Constant
  Display : Display
  Divide : Product  Inputs=**
  Divide1 : Product  Inputs=**
  Divide2 : Product  Inputs=*/
  Gain : Gain  Gain=1/15000
  Memory2 : Memory  X0=Theta_1_roll_last
  Mux : Mux  Inputs=12
  Roll Multilayer NN : MATLAB Function  TreatAsAtomicUnit=on
  Scope : Scope
      settings: YMin=-14  YMax=4  SaveName=ScopeData16
  Selector : Selector  InputPortWidth=3  Indices=3
  Terminator : Terminator
  Terminator1 : Terminator
  To Workspace : ToWorkspace  VariableName=Theta_1_roll_last  SampleTime=-1
      settings: MaxDataPoints=1
  To Workspace1 : ToWorkspace  VariableName=Theta_2_roll_last  SampleTime=-1
      settings: MaxDataPoints=1
  dem-less : Gain  Gain=T_sim
  v_ad_comp : Outport
  wires:
  p_chanel vars/1 -> Bus Selector1/1
  Bus Selector1/2 -> Mux/10  "<p_sf>"
  Bus Selector1/3 -> dem-less/1  "<p_sf_dot>"
  Bus Selector1/1 -> Mux/9, Roll Multilayer NN/2(e)  "<p_err>"
  Constant/1 -> Mux/1
  All_meas/1 -> Bus Selector2/1
  Bus Selector2/1 -> Gain/1  "<Alt meas (m)>"
  Divide/1 -> Mux/4
  Bus Selector2/3 -> Divide1/2, Divide1/1, Mux/5  "<AoA meas (rad)>"
  Divide1/1 -> Mux/6
  Bus Selector2/4 -> Mux/7  "<SS meas (rad)>"
  Gain/1 -> Mux/2
  Bus Selector2/5 -> Selector/1  "<omega_b meas (rad/s)>"
  Selector/1 -> Mux/8
  Roll Multilayer NN/1(v_ad_comp) -> v_ad_comp/1
  "   "/1 -> Roll Multilayer NN/8(Theta_2)
  B/1 -> Roll Multilayer NN/4(B)
  [P] -> Roll Multilayer NN/3(P)
  v_ad^ prev/1 -> Mux/12
  Roll Multilayer NN/4(Theta_1_update) -> To Workspace/1, Memory2/1
  Roll Multilayer NN/2(v_ad) -> Terminator/1
  Divide2/1 -> [P]
  Bus Selector1/4 -> Divide2/2  "<K_b_p>"
  Constant2/1 -> Divide2/1
  Bus Selector2/2 -> Divide/2, Divide/1, Mux/3  "<Mach>"
  Roll Multilayer NN/6(Theta_3_update) -> "  "/1, " "/1
  "  "/1 -> Roll Multilayer NN/9(Theta_3)
  Roll Multilayer NN/5(Theta_2_update) -> To Workspace1/1, "   "/1
  Memory2/1 -> Roll Multilayer NN/7(Theta_1)
  Roll_learning rate/1 -> Roll Multilayer NN/5(Roll_learnign_rate)
  Roll reg param/1 -> Roll Multilayer NN/6(Roll_reg_param)
  Mux/1 -> Display/1, Scope/1, Roll Multilayer NN/1(X_bar)
  Roll Multilayer NN/3(Z_norm_unit) -> Terminator1/1
  dem-less/1 -> Mux/11

== system lib_controller/Controller/NDI+CA Controller/4DOF ANN+NDI+CA Controller - No massic update/On-line (adaptive) multi-layer NNs/Yaw Channel/Yaw HL NN ==
  note: Be careful with dimensions of inputs!!!
      | NORMALIZATION!!!
  v_ad^ prev : Inport
  Yaw_chanel vars : Inport  Port=2
  All_meas : Inport  Port=3
  Yaw_learning rate : Inport  Port=4
  Yaw reg param : Inport  Port=5
  Bus Selector1 : BusSelector  OutputSignals=beta_chanel vars.beta_err,r_chanel vars.r_err,beta_chanel vars.beta_sf,beta_chanel vars.beta_sf_dot,r_chanel vars.r_sf_dot,beta_chanel vars.K_b_beta,r_chanel vars.K_b_r
  Bus Selector2 : BusSelector  OutputSignals=signal1.Alt meas (m),signal2.Mach,signal1.AoA meas (rad),signal1.Euler meas (rad)
  Constant : Constant
  Constant1 : Constant  Value=[0;1]
  Display : Display
  Divide : Product  Inputs=**
  Gain : Gain  Gain=1/15000
  Memory2 : Memory  X0=V_yaw_last
  Memory3 : Memory  X0=W_yaw_last
  Mux : Mux  Inputs=12
  Mux1 : Mux  Inputs=2
  Mux2 : Mux  Inputs=2
  Scope : Scope
      settings: YMin=-0.25  YMax=3.75  SaveName=ScopeData17
  Selector : Selector  InputPortWidth=3
  Terminator : Terminator
  Terminator1 : Terminator
  To Workspace : ToWorkspace  VariableName=V_yaw_last  SampleTime=-1
      settings: MaxDataPoints=1
  To Workspace1 : ToWorkspace  VariableName=W_yaw_last  SampleTime=-1
      settings: MaxDataPoints=1
  Yaw NN : MATLAB Function  TreatAsAtomicUnit=on
  dem-less1 : Gain  Gain=T_sim
  dem-less2 : Gain  Gain=T_sim^2
  v_ad_comp : Outport
  wires:
  Mux2/1 -> [Ks]
  Bus Selector1/6 -> Mux2/1  "<K_b_beta>"
  Bus Selector1/7 -> Mux2/2  "<K_b_r>"
  Mux1/1 -> Yaw NN/2(e)  "e"
  Divide/1 -> Mux/4
  Bus Selector2/1 -> Gain/1  "<Alt meas (m)>"
  All_meas/1 -> Bus Selector2/1
  Constant/1 -> Mux/1
  Yaw reg param/1 -> Yaw NN/6(Long_reg_param)
  Yaw_learning rate/1 -> Yaw NN/5(Long_learnign_rate)
  Yaw_chanel vars/1 -> Bus Selector1/1
  Yaw NN/1(v_ad_comp) -> v_ad_comp/1
  Yaw NN/4(W_update) -> Memory3/1, To Workspace1/1
  Memory2/1 -> Yaw NN/8(V)
  Memory3/1 -> Yaw NN/7(W)
  Constant1/1 -> Yaw NN/4(B)
  [Ks] -> Yaw NN/3(Ks)
  v_ad^ prev/1 -> Mux/12
  Yaw NN/5(V_update) -> Memory2/1, To Workspace/1
  Yaw NN/2(v_ad) -> Terminator/1
  Bus Selector2/4 -> Selector/1  "<Euler meas (rad)>"
  Gain/1 -> Mux/2
  Bus Selector2/2 -> Divide/2, Divide/1, Mux/3  "<Mach>"
  Bus Selector2/3 -> Mux/5  "<AoA meas (rad)>"
  Selector/1 -> Mux/6
  Bus Selector1/5 -> dem-less2/1  "<r_sf_dot>"
  Bus Selector1/2 -> Mux1/2, Mux/8  "<r_err>"
  Bus Selector1/4 -> dem-less1/1  "<beta_sf_dot>"
  Bus Selector1/1 -> Mux1/1, Mux/7  "<beta_err>"
  Bus Selector1/3 -> Mux/9  "<beta_sf>"
  Mux/1 -> Display/1, Scope/1, Yaw NN/1(X_bar)
  Yaw NN/3(Z_norm_unit) -> Terminator1/1
  dem-less1/1 -> Mux/10
  dem-less2/1 -> Mux/11

== matlab function lib_controller/Controller/NDI+CA Controller/9DOF NDI+CA Controller/DCM Arm1 ==
  data: eta input; T_Fb_FA output; gamma input
function T_Fb_FA = DCM_Arm(eta, gamma)
    % Rotation matrix from body to arm 1
    % Varm = R_B2Arm * Vbody
    T_Fb_FA = [ cos(gamma), sin(eta)*sin(gamma), -cos(eta)*sin(gamma);...
            0,cos(eta),sin(eta);...
            sin(gamma),-cos(gamma)*sin(eta),cos(gamma)*cos(eta) ];

== matlab function lib_controller/Controller/NDI+CA Controller/9DOF NDI+CA Controller/DCM Arm2 ==
  data: eta input; T_Fb_FA output; gamma input
function T_Fb_FA = DCM_Arm(eta, gamma)
    % Rotation matrix from body to arms 2 and 3
    % Varm = R_B2Arm * Vbody
    T_Fb_FA = [cos(eta),0,-sin(eta) ;...
            sin(eta)*sin(gamma),cos(gamma),cos(eta)*sin(gamma);...
            sin(eta)*cos(gamma),-sin(gamma),cos(eta)*cos(gamma)];

== matlab function lib_controller/Controller/NDI+CA Controller/9DOF NDI+CA Controller/DCM Arm3 ==
  data: eta input; T_Fb_FA output; gamma input
function T_Fb_FA = DCM_Arm(eta, gamma)
    % Rotation matrix from body to arms 2 and 3
    % Varm = R_B2Arm * Vbody
    T_Fb_FA = [cos(eta),0,-sin(eta) ;...
            sin(eta)*sin(gamma),cos(gamma),cos(eta)*sin(gamma);...
            sin(eta)*cos(gamma),-sin(gamma),cos(eta)*cos(gamma)];
